simulink model "CntIntgr1"  (Simulink 8.5)
settings: Solver=ode45  StartTime=0.0  StopTime=512  RelTol=1e-3
values from neighbouring files (symbols this model uses):
  k1 = 0.1    [init.m]
  kf = 0.1    [init.m]
libraries: simulink x1
settings Model: Creator=martin  LastModifiedBy=martin
settings DataIOCC: SignalLoggingSaveFormat=Dataset
settings OptimizationCC: ExpressionDepthLimit=128
settings DebuggingCC: UnderspecifiedInitializationDetection=Simplified  MergeDetectMultiDrivingBlocksExec=error  FcnCallInpInsideContextMsg=EnableAllAsError  StateNameClashWarn=none
settings GRTTargetCC: CombineOutputUpdateFcns=on  GRTInterface=off

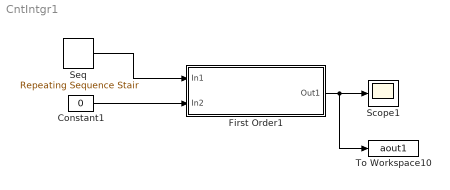
== system CntIntgr1 ==
  Constant1 : Constant  Value=0
  First Order1 : Subsystem  mask{k1=k1, k2=0, kf=kf}
      mask Display:
      | disp(sprintf('k1 = %0.6g\nk2 = %0.6g\nkf = %0.6g', ...
      |     k1, k2, kf));
  Scope1 : Scope
      settings: TimeRange=511  YMin=0  YMax=1  MaxDataPoints=2000000  SampleInput=on  SampleTime=Ts
  Seq : simulink/Sources/Repeating Sequence Stair  OutValues=dat  tsamp=Ts  OutMin=[]  OutMax=[]  OutDataTypeStr=double  OutputDataTypeScalingMode=double  OutDataType=fixdt(0,8)  ConRadixGroup=Best Precision: Vector-wise  OutScaling=2^-12  mask(Repeating Sequence Stair){}
  To Workspace10 : ToWorkspace  VariableName=aout1  SampleTime=-1
      settings: MaxDataPoints=128*16 - 1
  wires:
  Seq/1 -> First Order1/1(In1)
  Constant1/1 -> First Order1/2(In2)
  First Order1/1(Out1) -> To Workspace10/1, Scope1/1

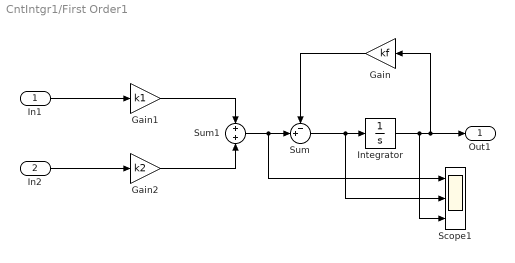
== system CntIntgr1/First Order1 ==
  In1 : Inport
  In2 : Inport  Port=2
  Gain : Gain  Gain=kf
  Gain1 : Gain  Gain=k1
  Gain2 : Gain  Gain=k2
  Integrator : Integrator
  Scope1 : Scope  NumInputPorts=3
      settings: TimeRange=511  YMin=0~-5~-5  YMax=1~5~5  MaxDataPoints=2000000  SampleInput=on  SampleTime=Ts
  Sum : Sum  Inputs=-+|
  Sum1 : Sum  Inputs=+|+
  Out1 : Outport
  wires:
  Integrator/1 -> Scope1/3, Gain/1, Out1/1
  Gain1/1 -> Sum1/1
  Gain2/1 -> Sum1/2
  In2/1 -> Gain2/1
  Sum1/1 -> Scope1/1, Sum/2
  In1/1 -> Gain1/1
  Gain/1 -> Sum/1
  Sum/1 -> Scope1/2, Integrator/1
